simulink model "SimulateLidarSensor_Highway"  (R2020a)
settings: Solver=VariableStepAuto  StartTime=0.0  StopTime=50  RelTol=1e-3
PreLoadFcn:
  | % Load reference path for recorded drive segment
  | data = load('sim3d_DriveSegmentUSCityBlock.mat');
  | 
  | % Setup workspace variables used by model
  | refPosesX = data.driveSegmentUSCityBlock.refPathX;
  | refPosesY = data.driveSegmentUSCityBlock.refPathY;
  | refPosesT = data.driveSegmentUSCityBlock.refPathT;
  | 
  | % Set mode to record only
  | recordMode = true;
values from neighbouring files (symbols this model uses):
  trajectory =     [Realistic_trajectory1.mat]    (also in Realistic_trajectory2.mat; Realistic_trajectory3.mat; Realistic_trajectory4.mat; Realistic_trajectory5.mat)
libraries: sim3dautolib x2, sim3dphyssensorlib x1, sim3dlib x1
settings Model: Creator=The MathWorks, Inc.  LastModifiedBy=M-Mpwo
settings DebuggingCC: SymbolicDimsDataTypeCodeGenerationDiagnostic=none

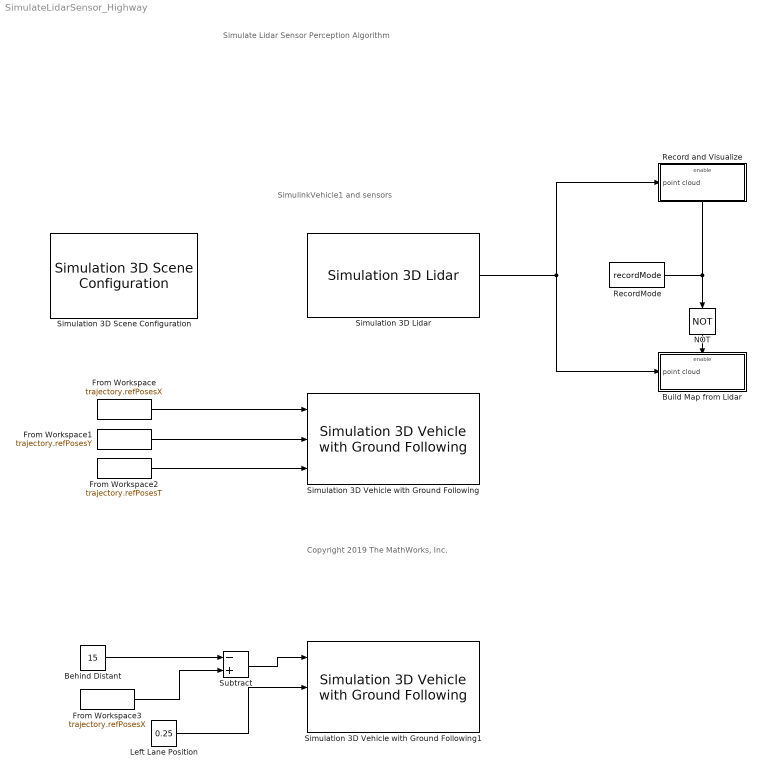
== system SimulateLidarSensor_Highway ==
  note: Simulate Lidar Sensor Perception Algorithm
  note: SimulinkVehicle1 and sensors
  note: Copyright 2019 The MathWorks, Inc.
  Behind Distant : Constant  Value=15
  Build Map from Lidar : Subsystem  TreatAsAtomicUnit=on
  From Workspace : FromWorkspace  VariableName=trajectory.refPosesX  OutputAfterFinalValue=Holding final value
  From Workspace1 : FromWorkspace  VariableName=trajectory.refPosesY  OutputAfterFinalValue=Holding final value
  From Workspace2 : FromWorkspace  VariableName=trajectory.refPosesT  OutputAfterFinalValue=Holding final value
  From Workspace3 : FromWorkspace  VariableName=trajectory.refPosesX  OutputAfterFinalValue=Holding final value
  Left Lane Position : Constant  Value=0.25
  NOT : Logic  Operator=NOT  IconShape=distinctive  AllPortsSameDT=off  OutDataTypeStr=boolean
  Record and Visualize : Subsystem  TreatAsAtomicUnit=on
  RecordMode : Constant  Value=recordMode
  Simulation 3D Lidar : sim3dphyssensorlib/Simulation 3D Lidar  sensorTag=Sim3dSensor1  sensorId=1  sensorName=Sim3dSensor1  vehTagList={'Scene Origin';'SimulinkVehicle1'}  vehTag=Scene Origin  mountLoc=Origin  offsetFlag=on  tmountOffset=[400, -4.5, 3]  rmountOffset=[0, 0, 0]  DetectionRange=90  RangeResolution=0.002  VerticalFOV=40  VerticalResolution=1.25  HorizontalFOV=360  HorizontalResolution=0.332409972299169  DistanceOutportEnabled=off  TransformOutportEnabled=off  SampleTime=-1  mountPoint=[400 4.5 3]  mountOrientation=[0 0 0]  aMode=3  ID=1
      settings: SourceProductBaseCode=DR,VE
  Simulation 3D Scene Configuration : sim3dlib/Simulation 3D Scene Configuration  Priority=0  ProjectFormat=Unreal Executable  SceneDesc=Straight road  ProjectName=C:\Users\m-Mpwo\Documents\Unreal_Maps\WindowsNoEditor\AutoVrtlEnv.exe  ScenePath=/Game/Maps/HwStrght  UEProjPath=C:\Local\AutoVrtlEnv\AutoVrtlEnv.uproject  vehTagList={'Scene Origin';'SimulinkVehicle1'}  vehTag=SimulinkVehicle1  OpVisEn=off  Ts=1/60  EnableWindow=on  sensorTag=MainCamera1  sensorId=1  sensorName=MainCamera1  mountLoc=Origin  offsetFlag=off  tmountOffset=[0, 0, 0]  rmountOffset=[0, 0, 0]  HorizontalResolution=1280  VerticalResolution=720  HorizontalFOV=60  mountPoint=[0 0 0]  mountOrientation=[0 0 0]  aMode=3  ID=1
      settings: SourceProductBaseCode=DR,VE
  Simulation 3D Vehicle with Ground Following : sim3dautolib/Simulation 3D Vehicle with Ground Following  Priority=-1  PassVehMesh=Hatchback  VehColor=Red  InitialPos=[trajectory.refPosesX(1,2), trajectory.refPosesY(1,2), 0]  InitialRot=[0, 0, trajectory.refPosesT(1,2)]  ActorName=SimulinkVehicle1  SampleTime=-1  ActorType=SimulinkVehicle  ID=1  aMode=3  ActorTag=SimulinkVehicle1  CoordinateScheme=ISO  TransformOutportEnabled=off
      settings: SourceProductBaseCode=DR,VE
  Simulation 3D Vehicle with Ground Following1 : sim3dautolib/Simulation 3D Vehicle with Ground Following  Priority=-1  PassVehMesh=Hatchback  VehColor=Green  InitialPos=[trajectory.refPosesX(1,2), trajectory.refPosesY(1,2), 0]  InitialRot=[0, 0, trajectory.refPosesT(1,2)]  ActorName=SimulinkVehicle2  SampleTime=-1  ActorType=SimulinkVehicle  ID=2  aMode=3  ActorTag=SimulinkVehicle2  CoordinateScheme=ISO  TransformOutportEnabled=off
      settings: SourceProductBaseCode=DR,VE
  Subtract : Sum  Inputs=-+
  wires:
  From Workspace2/1 -> Simulation 3D Vehicle with Ground Following/3
  From Workspace1/1 -> Simulation 3D Vehicle with Ground Following/2
  From Workspace/1 -> Simulation 3D Vehicle with Ground Following/1
  Simulation 3D Lidar/1 -> Build Map from Lidar/1(point cloud), Record and Visualize/1(point cloud)
  RecordMode/1 -> NOT/1, Record and Visualize/Enable
  NOT/1 -> Build Map from Lidar/Enable
  From Workspace3/1 -> Subtract/2
  Behind Distant/1 -> Subtract/1
  Subtract/1 -> Simulation 3D Vehicle with Ground Following1/1
  Left Lane Position/1 -> Simulation 3D Vehicle with Ground Following1/2

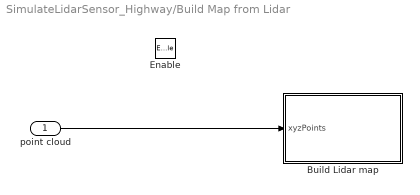
== system SimulateLidarSensor_Highway/Build Map from Lidar ==
  point cloud : Inport
  Enable : EnablePort
  Build Lidar map : MATLAB Function  TreatAsAtomicUnit=on
  wires:
  point cloud/1 -> Build Lidar map/1(xyzPoints)

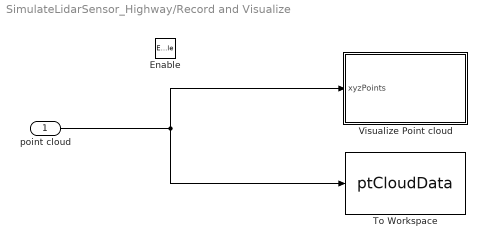
== system SimulateLidarSensor_Highway/Record and Visualize ==
  point cloud : Inport
  Enable : EnablePort
  To Workspace : ToWorkspace  VariableName=ptCloudData  SaveFormat=Structure With Time  SampleTime=-1
  Visualize Point cloud : MATLAB Function  StopFcn=|  TreatAsAtomicUnit=on
      | playerFigure = findall(groot,'type','figure','name','Point Cloud Player');
      | 
      | if ~isempty(playerFigure)
      |     playerFigure = playerFigure(end);
      |     if isvalid(playerFigure)
      |         close(playerFigure);
      |     end
      | end
  wires:
  point cloud/1 -> To Workspace/1, Visualize Point cloud/1(xyzPoints)

== matlab function SimulateLidarSensor_Highway/Record and Visualize/Visualize Point cloud ==
  data: xyzPoints input
function VisualizePointCloud(xyzPoints)
%VisualizePointCloud Display point cloud

coder.extrinsic('isOpen', 'pcplayer')

persistent player;

if isempty(player)
    % Configure axes limits
    xlimits = [-90 90];
    ylimits = [-90 90];
    zlimits = [ -90 90];
    
    % Create a streaming Lidar viewer
    player = pcplayer(xlimits, ylimits, zlimits);
end

if ~isempty(player) && isOpen(player)
    view(player, xyzPoints);
end

== matlab function SimulateLidarSensor_Highway/Build Map from Lidar/Build Lidar map ==
  data: xyzPoints input
function buildLidarMap(xyzPoints)
%buildLidarMap Build a map from Lidar data

coder.extrinsic('pointCloud', 'helperLidarMapBuilder', 'updateMap', 'updateDisplay')

persistent mapBuilder frameCount

% Number of frames to skip between successive map updates
skipFrames = 5;

% Create a map builder object
if isempty(mapBuilder)
    mapBuilder = helperLidarMapBuilder;
end

% Initialize frame count
if isempty(frameCount)
    frameCount = 1;
end

% Increment frameCount
frameCount = frameCount + 1;

closeDisplay = false;

if mod(frameCount-1, skipFrames)==0
    % Create a pointCloud object from point locations
    ptCloud = pointCloud(xyzPoints);
    
    % Update map with new pointCloud
    updateMap(mapBuilder, ptCloud);
    
    updateDisplay(mapBuilder, closeDisplay);
end
end
